simulink model "MPC_sim_switch"  (R2017b)
settings: Solver=VariableStepAuto  StartTime=0.0  StopTime=4  RelTol=1e-3
libraries: simulink x2, mpclib x1, dspmtrx3 x1
settings Model: Creator=pimwu  LastModifiedBy=pimwu
settings OptimizationCC: LifeSpan=inf
settings DebuggingCC: SFExecutionAtInitializationDiag=none
settings CodeAppCC: StateflowObjectComments=on

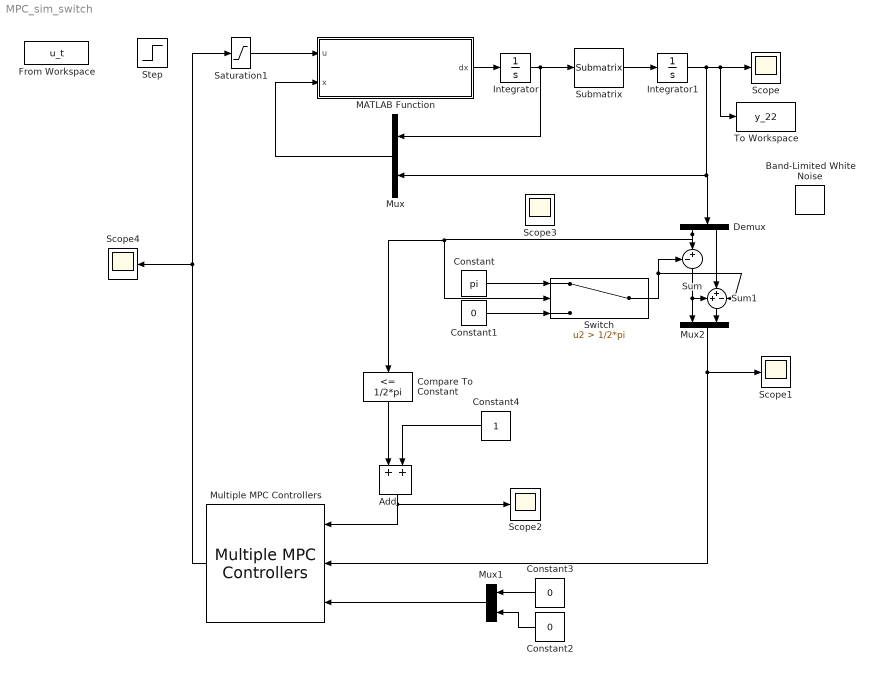
== system MPC_sim_switch ==
  Add : Sum
  Band-Limited White Noise : simulink/Sources/Band-Limited White Noise  Cov=[0.00000003]  Ts=0.002  seed=[23341]
  Compare To Constant : simulink/Logic and Bit Operations/Compare To Constant  relop=<=  const=1/2*pi  OutDataTypeStr=boolean
  Constant : Constant  Value=pi
  Constant1 : Constant  Value=0
  Constant2 : Constant  Value=0
  Constant3 : Constant  Value=0
  Constant4 : Constant
  Demux : Demux  Outputs=2
  From Workspace : FromWorkspace  VariableName=u_t  SampleTime=0
  Integrator : Integrator  InitialCondition=[0 0 0]
  Integrator1 : Integrator  InitialCondition=[pi;pi+0.02]
  MATLAB Function : MATLAB Function  TreatAsAtomicUnit=on
  Multiple MPC Controllers : mpclib/Multiple MPC Controllers  mpcobjs="{'MPCpi0','MPC_00'  }"  x0s={'[]','[]' }  Nmpc=1  theMPC=1  nmv=1  nmo=1  nmd=1  nts=1  is_designfromscratch=0  linswitch=0  ref_from_ws_multiple=off  ref_signal_name_multiple=[]  ref_preview_multiple=off  md_from_ws_multiple=off  md_signal_name_multiple=[]  md_preview_multiple=off  md_inport_multiple=off  mv_inport_multiple=off  cost_outport_multiple=off  return_sequence_multiple=off  return_qpstatus_multiple=off  return_state_multiple=off  state_inport_multiple=off  lims_inport_multiple=off  ywt_inport_multiple=off  uwt_inport_multiple=off  duwt_inport_multiple=off  rhoeps_inport_multiple=off  uref_inport_multiple=off  BlockDataType_multiple=double  SampleTimeInherited_multiple=off
      settings: SourceProductName=Model Predictive Control Toolbox  SourceProductBaseCode=MP
  Mux : Mux  Inputs=2
  Mux1 : Mux  Inputs=2
  Mux2 : Mux  Inputs=2
  Saturation1 : Saturate  UpperLimit=1  LowerLimit=-1
  Scope{,1..4} (5 alike) : Scope
  Step : Step  Time=0  After=-1  SampleTime=0
  Submatrix : dspmtrx3/Submatrix  RowSpan=Range of rows  RowStartMode=First  RowStartIndex=1  RowEndMode=Index  RowEndIndex=2  ColSpan=Range of columns  ColStartMode=First  ColStartIndex=1  ColEndMode=Last  ColEndIndex=1
  Sum : Sum  Inputs=-+|
  Sum1 : Sum  Inputs=++-
  Switch : Switch  Criteria=u2 > Threshold  Threshold=1/2*pi
  To Workspace : ToWorkspace  VariableName=y_22  SaveFormat=Timeseries  SampleTime=-1
  wires:
  MATLAB Function/1(dx) -> Integrator/1
  Integrator/1 -> Submatrix/1, Mux/1
  Submatrix/1 -> Integrator1/1
  Mux/1 -> MATLAB Function/2(x)
  Saturation1/1 -> MATLAB Function/1(u)
  Sum/1 -> Sum1/1, Mux2/1
  Sum1/1 -> Mux2/2
  Demux/2 -> Sum1/2
  Demux/1 -> Compare To Constant/1, Switch/2, Sum/2
  Add/1 -> Scope2/1, Multiple MPC Controllers/1
  Mux2/1 -> Scope1/1, Multiple MPC Controllers/2
  Mux1/1 -> Multiple MPC Controllers/3
  Constant4/1 -> Add/2
  Compare To Constant/1 -> Add/1
  Integrator1/1 -> To Workspace/1, Scope/1, Demux/1, Mux/2
  Constant/1 -> Switch/1
  Constant1/1 -> Switch/3
  Constant3/1 -> Mux1/1
  Constant2/1 -> Mux1/2
  Multiple MPC Controllers/1 -> Saturation1/1, Scope4/1
  Switch/1 -> Sum1/3, Sum/1

== matlab function MPC_sim_switch/MATLAB Function ==
  data: u input; x input; dx output
function dx = nonlinsim_interpreted(u,x)
theta1  = x(4);
theta2  = x(5);
theta1d = x(1);
theta2d = x(2);
ii      = x(3);
par =     [0.107001615392530   0.165343973632010   0.040783104942133   0.046364080778153   0.000051655820835   0.048856187724916   0.049137116812930   1.636038234993470   0.000031810472615   1.827977549139487   0.000008590269497   0.006045619229031   3.032790298604742   0.098524631245120   1.049678153165582];

%Define parameters
L1 = par(1);m1 = par(2);m2 = par(3); I1 = par(4); I2 = par(5);
c1 = par(6); c2 = par(7); 
b1 = par(8); b2 = par(9);  Bc1 = par(10); Bc2 = par(11);
 L = par(12); Kt = par(13); R = par(14); Kv = par(15);
g = 9.81;
M = -7;
%Input
Tau = u;%interp1(u.Time,u.Data,t);
dx = zeros(3,1);
% dx(1) = x(3);
% dx(2) = x(4);
dx(1) = (3*I2*Kt*ii - 2*Bc2*I2*atan(4*theta1d - 4*theta2d) - 2*Bc1*I2*atan(4*theta1d) - 3*I2*b1*theta1d - 3*I2*b2*theta1d + 3*I2*b2*theta2d - 2*Bc1*c2^2*m2*atan(4*theta1d) - 4*Bc2*c2^2*m2*atan(4*theta1d - 4*theta2d) + 3*Kt*c2^2*ii*m2 - 3*b1*c2^2*m2*theta1d - 6*b2*c2^2*m2*theta1d + 6*b2*c2^2*m2*theta2d + 3*L1*c2^2*g*m2^2*sin(theta1) + 3*I2*c2*g*m2*sin(theta1 + theta2) + 3*I2*L1*g*m2*sin(theta1) + 3*I2*c1*g*m1*sin(theta1) + 3*L1*c2^3*m2^2*theta1d^2*sin(theta2) + 3*L1*c2^3*m2^2*theta2d^2*sin(theta2) + 6*L1*c2^3*m2^2*theta1d*theta2d*sin(theta2) - 3*L1*b2*c2*m2*theta1d*cos(theta2) + 3*L1*b2*c2*m2*theta2d*cos(theta2) + 3*L1^2*c2^2*m2^2*theta1d^2*cos(theta2)*sin(theta2) - 3*L1*c2^2*g*m2^2*sin(theta1 + theta2)*cos(theta2) + 3*I2*L1*c2*m2*theta2d^2*sin(theta2) + 3*c1*c2^2*g*m1*m2*sin(theta1) - 2*Bc2*L1*c2*m2*atan(4*theta1d - 4*theta2d)*cos(theta2) + 6*I2*L1*c2*m2*theta1d*theta2d*sin(theta2))/(3*(I1*I2 + L1^2*c2^2*m2^2 + I2*L1^2*m2 + I1*c2^2*m2 + I2*c2^2*m2 - L1^2*c2^2*m2^2*cos(theta2)^2 + 2*I2*L1*c2*m2*cos(theta2)));
dx(2) =  -(3*I1*b2*theta2d - 3*I1*b2*theta1d - 2*Bc2*I1*atan(4*theta1d - 4*theta2d) - 2*Bc1*c2^2*m2*atan(4*theta1d) - 2*Bc2*L1^2*m2*atan(4*theta1d - 4*theta2d) - 4*Bc2*c2^2*m2*atan(4*theta1d - 4*theta2d) + 3*Kt*c2^2*ii*m2 - 3*L1^2*b2*m2*theta1d + 3*L1^2*b2*m2*theta2d - 3*b1*c2^2*m2*theta1d - 6*b2*c2^2*m2*theta1d + 6*b2*c2^2*m2*theta2d - 3*L1^2*c2*g*m2^2*sin(theta1 + theta2) + 3*L1*c2^2*g*m2^2*sin(theta1) - 3*I1*c2*g*m2*sin(theta1 + theta2) + 3*L1*c2^3*m2^2*theta1d^2*sin(theta2) + 3*L1^3*c2*m2^2*theta1d^2*sin(theta2) + 3*L1*c2^3*m2^2*theta2d^2*sin(theta2) + 3*Kt*L1*c2*ii*m2*cos(theta2) + 6*L1*c2^3*m2^2*theta1d*theta2d*sin(theta2) - 3*L1*b1*c2*m2*theta1d*cos(theta2) - 9*L1*b2*c2*m2*theta1d*cos(theta2) + 9*L1*b2*c2*m2*theta2d*cos(theta2) + 6*L1^2*c2^2*m2^2*theta1d^2*cos(theta2)*sin(theta2) + 3*L1^2*c2^2*m2^2*theta2d^2*cos(theta2)*sin(theta2) - 3*L1*c2^2*g*m2^2*sin(theta1 + theta2)*cos(theta2) + 3*L1^2*c2*g*m2^2*cos(theta2)*sin(theta1) + 3*I1*L1*c2*m2*theta1d^2*sin(theta2) + 3*c1*c2^2*g*m1*m2*sin(theta1) - 2*Bc1*L1*c2*m2*atan(4*theta1d)*cos(theta2) - 6*Bc2*L1*c2*m2*atan(4*theta1d - 4*theta2d)*cos(theta2) + 6*L1^2*c2^2*m2^2*theta1d*theta2d*cos(theta2)*sin(theta2) + 3*L1*c1*c2*g*m1*m2*cos(theta2)*sin(theta1))/(3*(I1*I2 + L1^2*c2^2*m2^2 + I2*L1^2*m2 + I1*c2^2*m2 + I2*c2^2*m2 - L1^2*c2^2*m2^2*cos(theta2)^2 + 2*I2*L1*c2*m2*cos(theta2)));
dx(3) = -(R*ii - M*Tau + Kv*theta1d)/L;
% dx = dx';

end
